simulink model "modello_simulink"  (R2019b)
settings: Solver=VariableStepAuto  StartTime=0.0  StopTime=300.0  RelTol=1e-3
values from neighbouring files (symbols this model uses):
  a1 = rho * D^4 * alpha1    (= 0.000388302366464)    [data.m]    (also in simout.mat)
  a2 = -rho * D^3 * alpha2 * (1 - omega)    (= 0.0037030698432)    [data.m]    (also in simout.mat)
  alpha1 = 0.0113    [data.m]    (also in simout.mat)
  alpha2 = -0.0091    [data.m]    (also in simout.mat)
  current = [seaCurrent; 0; 0; 0]    [data.m]    (also in simout.mat = [0 0 0 0 0 0])
  D = diag([])    [D.m]    (also in data.m = 0.076; simout.mat = 0.076)
  dead_zone_limit = 31.5    [data.m]    (also in simout.mat)
  initial = [0 0 0 0 0 0]'    [Plot_verifica_modello.m]    (also in data.m = [0;0;0;0;0;0]; simout.mat = [0 0 0 0 0 0])
  M = [67.0334425707 0 0 0 0 0 0 67.0334425707 0 0 0 0 ... (36 elements, 6x6)]    [M.mat]    (also in Masse.m = M_rb + M_a; simout.mat)
  M_inv = inv(M)    [Masse.m]    (also in simout.mat = [0.0149179269578 0 0 0 0 0 0 0.0149179269578 0 0 0 0 ... (36)
  n_max = 340    [data.m]    (also in simout.mat)
  omega = 0.1    [data.m]    (also in simout.mat)
  pylonCenter = [ 43.723046 ... (first row only)    [missionB.m]    (also in simout.mat = [43.723046 10.396635 0])
  rho = 1030    [data.m]    (also in simout.mat)
  TAM = [B1 B2 B3 B4 B5 B6 B7]    [TAM_matrice.m]    (also in simout.mat = [1 0 0 0 0 0.25 1 0 0 0 0 -0.25 ... (42 elements, 6x7)])
settings Model: Creator=andrea  LastModifiedBy=Fabio
settings DebuggingCC: ArithmeticOperatorsInVariantConditions=warning
settings SFSimCC: CustomCodeUndefinedFunction=UseInterfaceOnly

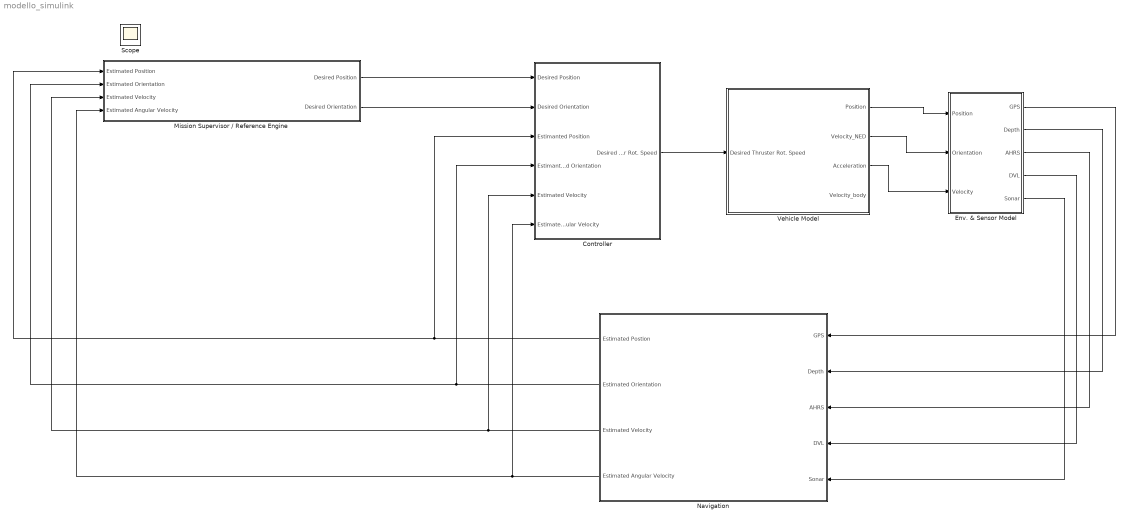
== system modello_simulink ==
  Controller : Subsystem
  Env. & Sensor Model : Subsystem
  Mission Supervisor / Reference Engine : Subsystem
  Navigation : Subsystem
  Vehicle Model : Subsystem
      mask Display: image('maronn.jpg'); % Use "Edit Image" on toolstrip to change.
  Scope : Scope
  wires:
  Mission Supervisor / Reference Engine/1(Desired Position) -> Controller/1(Desired Position)
  Mission Supervisor / Reference Engine/2(Desired Orientation) -> Controller/2(Desired Orientation)
  Controller/1(Desired Thruster Rot. Speed) -> Vehicle Model/1(Desired Thruster Rot. Speed)
  Vehicle Model/1(Position) -> Env. & Sensor Model/1(Position)
  Vehicle Model/2(Velocity_NED) -> Env. & Sensor Model/2(Orientation)
  Vehicle Model/3(Acceleration) -> Env. & Sensor Model/3(Velocity)
  Env. & Sensor Model/1(GPS) -> Navigation/1(GPS)
  Env. & Sensor Model/2(Depth) -> Navigation/2(Depth)
  Env. & Sensor Model/3(AHRS) -> Navigation/3(AHRS)
  Env. & Sensor Model/4(DVL) -> Navigation/4(DVL)
  Env. & Sensor Model/5(Sonar) -> Navigation/5(Sonar)
  Navigation/1(Estimated Postion) -> Controller/3(Estimanted Position), Mission Supervisor / Reference Engine/1(Estimated Position)
  Navigation/2(Estimated Orientation) -> Mission Supervisor / Reference Engine/2(Estimated Orientation), Controller/4(Estimanted Orientation)
  Navigation/3(Estimated Velocity) -> Mission Supervisor / Reference Engine/3(Estimated Velocity), Controller/5(Estimated Velocity)
  Navigation/4(Estimated Angular Velocity) -> Mission Supervisor / Reference Engine/4(Estimated Angular Velocity), Controller/6(Estimated Angular Velocity)

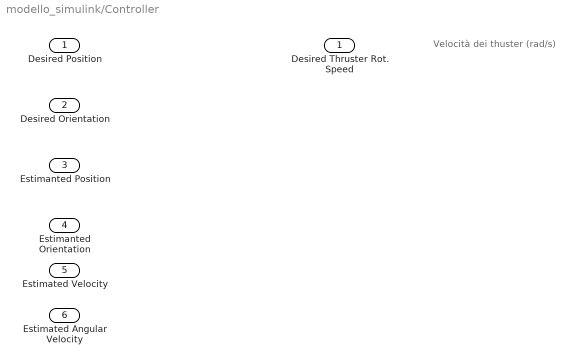
== system modello_simulink/Controller ==
  note: Velocità dei thuster (rad/s)
  Desired Position : Inport
  Desired Orientation : Inport  Port=2
  Estimanted Position : Inport  Port=3
  Estimanted Orientation : Inport  Port=4
  Estimated Velocity : Inport  Port=5
  Estimated Angular Velocity : Inport  Port=6
  Desired Thruster Rot. Speed : Outport

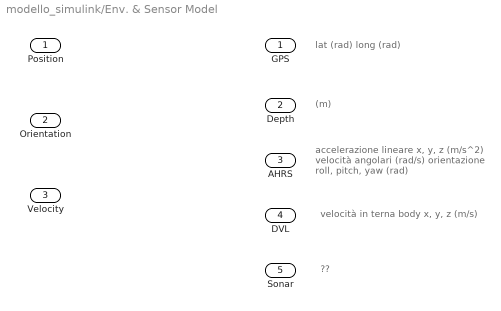
== system modello_simulink/Env. & Sensor Model ==
  note: ??
  note: velocità in terna body x, y, z (m/s)
  note: accelerazione lineare x, y, z (m/s^2)
      | velocità angolari (rad/s)
      | orientazione roll, pitch, yaw (rad)
  note: (m)
  note: lat (rad)
      | long (rad)
  Position : Inport
  Orientation : Inport  Port=2
  Velocity : Inport  Port=3
  GPS : Outport
  Depth : Outport  Port=2
  AHRS : Outport  Port=3
  DVL : Outport  Port=4
  Sonar : Outport  Port=5

== system modello_simulink/Mission Supervisor // Reference Engine ==
  note: Roll (rad): 0 == aligned with water surface
      | Pitch (rad): 0 == aligned with water surface
      | Yaw (rad): 0 == north
  note: Latitude (rad)
      | Longitude (rad)
      | Depth (m): 0 == water surface
  note: Latitude (rad)
      | Longitude (rad)
      | Depth (m): 0 == water surface
  note: Roll (rad): 0 == aligned with water surface
      | Pitch (rad): 0 == aligned with water surface
      | Yaw (rad): 0 == north
  note: Velocity body frame - x, y, z (m/s)
  note: Inertial Frame
      | Roll Rate (rad/s)
      | Pitch Rate (rad/s)
      | Yaw Rate (rad/s)
  Estimated Position : Inport
  Estimated Orientation : Inport  Port=2
  Estimated Velocity : Inport  Port=3
  Estimated Angular Velocity : Inport  Port=4
  Desired Position : Outport
  Desired Orientation : Outport  Port=2

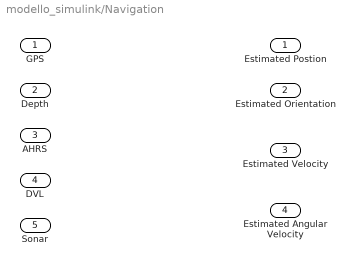
== system modello_simulink/Navigation ==
  GPS : Inport
  Depth : Inport  Port=2
  AHRS : Inport  Port=3
  DVL : Inport  Port=4
  Sonar : Inport  Port=5
  Estimated Postion : Outport
  Estimated Orientation : Outport  Port=2
  Estimated Velocity : Outport  Port=3
  Estimated Angular Velocity : Outport  Port=4

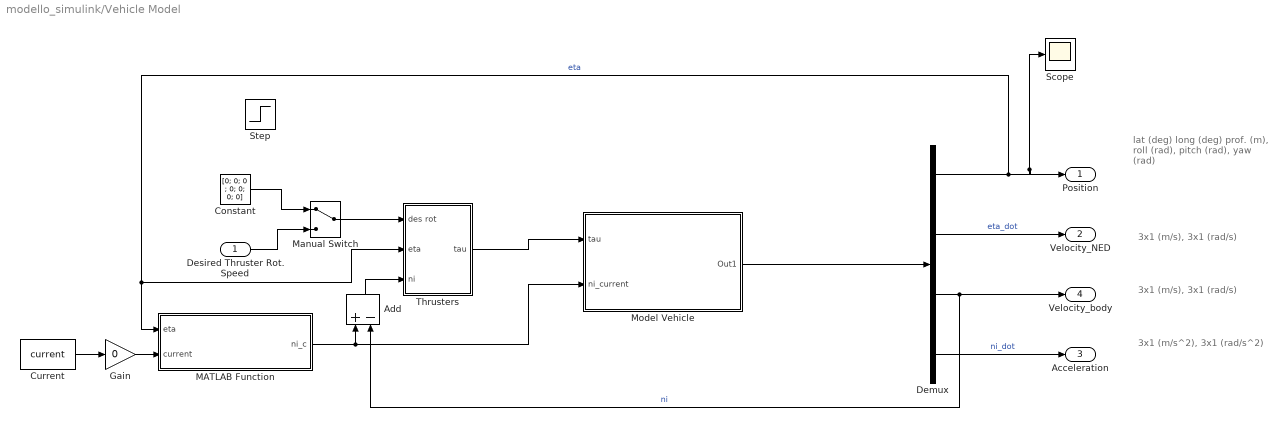
== system modello_simulink/Vehicle Model ==
  note: 3x1 (m/s^2),
      | 3x1 (rad/s^2)
  note: 3x1 (m/s),
      | 3x1 (rad/s)
  note: lat (deg)
      | long (deg)
      | prof. (m),
      | roll (rad),
      | pitch (rad),
      | yaw (rad)
  note: 3x1 (m/s),
      | 3x1 (rad/s)
  Desired Thruster Rot. Speed : Inport
  Add : Sum  Inputs=+-
  Constant : Constant  Value=[0; 0; 0 ; 0; 0; 0; 0]
  Current : Constant  Value=current
  Demux : Demux
  Gain : Gain  Gain=0
  MATLAB Function : MATLAB Function  TreatAsAtomicUnit=on
  Manual Switch : ManualSwitch
  Model Vehicle : Subsystem
      mask Display: image('anna.jpg'); % Use "Edit Image" on toolstrip to change.
  Scope : Scope
  Step : Step  Time=100  Before=[0;0;0;0;-100;-100;-200]  After=[0;0;0;0;0;0;0]  SampleTime=0
  Thrusters : Subsystem
  Position : Outport
  Velocity_NED : Outport  Port=2
  Acceleration : Outport  Port=3
  Velocity_body : Outport  Port=4
  wires:
  Demux/3 -> Velocity_body/1, Add/2  "ni"
  Model Vehicle/1(Out1) -> Demux/1
  Demux/1 -> Thrusters/2(eta), MATLAB Function/1(eta), Position/1, Scope/1  "eta"
  Desired Thruster Rot. Speed/1 -> Manual Switch/2
  Manual Switch/1 -> Thrusters/1(des rot)
  Current/1 -> Gain/1
  Gain/1 -> MATLAB Function/2(current)
  Demux/2 -> Velocity_NED/1  "eta_dot"
  Demux/4 -> Acceleration/1  "ni_dot"
  Thrusters/1(tau) -> Model Vehicle/1(tau)
  Constant/1 -> Manual Switch/1
  MATLAB Function/1(ni_c) -> Model Vehicle/2(ni_current), Add/1
  Add/1 -> Thrusters/3(ni)

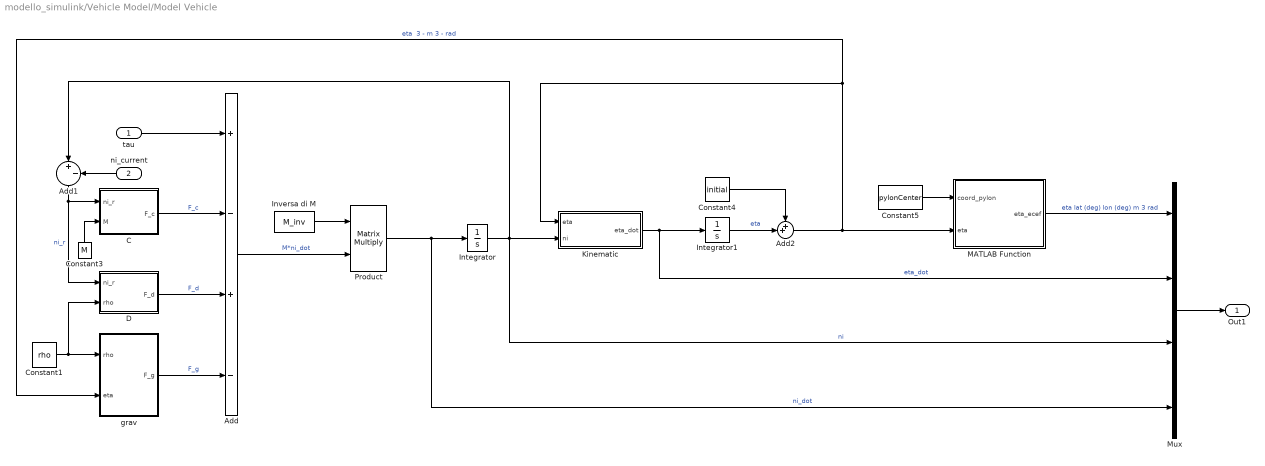
== system modello_simulink/Vehicle Model/Model Vehicle ==
  tau : Inport
  ni_current : Inport  Port=2
  Add : Sum  Inputs=+-+-
  Add1 : Sum  Inputs=|+-
  Add2 : Sum  Inputs=++|
  C : MATLAB Function  TreatAsAtomicUnit=on
  Constant1 : Constant  Value=rho
  Constant3 : Constant  Value=M
  Constant4 : Constant  Value=initial
  Constant5 : Constant  Value=pylonCenter
  D : MATLAB Function  TreatAsAtomicUnit=on
  Integrator : Integrator
  Integrator1 : Integrator
  Inversa di M : Constant  Value=M_inv
  Kinematic : Subsystem
  MATLAB Function : MATLAB Function  TreatAsAtomicUnit=on
  Mux : Mux
  Product : Product  Multiplication=Matrix(*)
  grav : MATLAB Function  TreatAsAtomicUnit=on
  Out1 : Outport  VectorParamsAs1DForOutWhenUnconnected=off
  wires:
  tau/1 -> Add/1
  Product/1 -> Mux/4, Integrator/1  "ni_dot"
  Integrator/1 -> Mux/3, Kinematic/2(ni), Add1/1  "ni"
  ni_current/1 -> Add1/2
  Add1/1 -> D/1(ni_r), C/1(ni_r)  "ni_r"
  Mux/1 -> Out1/1
  C/1(F_c) -> Add/2  "F_c"
  grav/1(F_g) -> Add/4  "F_g"
  Kinematic/1(eta_dot) -> Mux/2, Integrator1/1  "eta_dot"
  Inversa di M/1 -> Product/1
  Add/1 -> Product/2  "M*ni_dot"
  Constant1/1 -> grav/1(rho), D/2(rho)
  Constant3/1 -> C/2(M)
  D/1(F_d) -> Add/3  "F_d"
  Add2/1 -> MATLAB Function/2(eta), grav/2(eta), Kinematic/1(eta)  "eta  3 - m 3 - rad"
  MATLAB Function/1(eta_ecef) -> Mux/1  "eta lat (deg) lon (deg) m 3 rad"
  Constant5/1 -> MATLAB Function/1(coord_pylon)
  Constant4/1 -> Add2/1
  Integrator1/1 -> Add2/2  "eta"

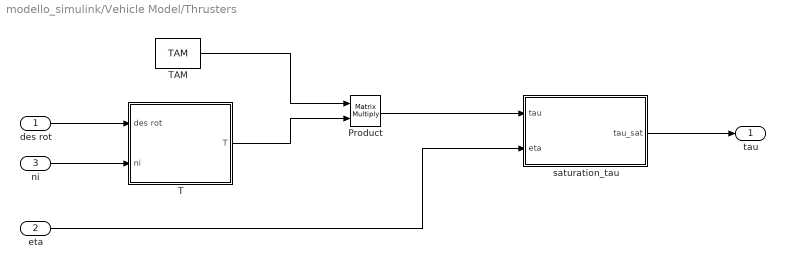
== system modello_simulink/Vehicle Model/Thrusters ==
  des rot : Inport
  eta : Inport  Port=2
  ni : Inport  Port=3
  Product : Product  Multiplication=Matrix(*)
  T : Subsystem
  TAM : Constant  Value=TAM
  saturation_tau : MATLAB Function  TreatAsAtomicUnit=on
  tau : Outport  VectorParamsAs1DForOutWhenUnconnected=off
  wires:
  Product/1 -> saturation_tau/1(tau)
  des rot/1 -> T/1(des rot)
  TAM/1 -> Product/1
  T/1(T) -> Product/2
  saturation_tau/1(tau_sat) -> tau/1
  ni/1 -> T/2(ni)
  eta/1 -> saturation_tau/2(eta)

== system modello_simulink/Vehicle Model/Model Vehicle/Kinematic ==
  eta : Inport
  ni : Inport  Port=2
  Jac : MATLAB Function  TreatAsAtomicUnit=on
  Product : Product  Multiplication=Matrix(*)
  eta_dot : Outport  VectorParamsAs1DForOutWhenUnconnected=off
  wires:
  ni/1 -> Product/2
  Jac/1(J) -> Product/1
  eta/1 -> Jac/1(eta)
  Product/1 -> eta_dot/1

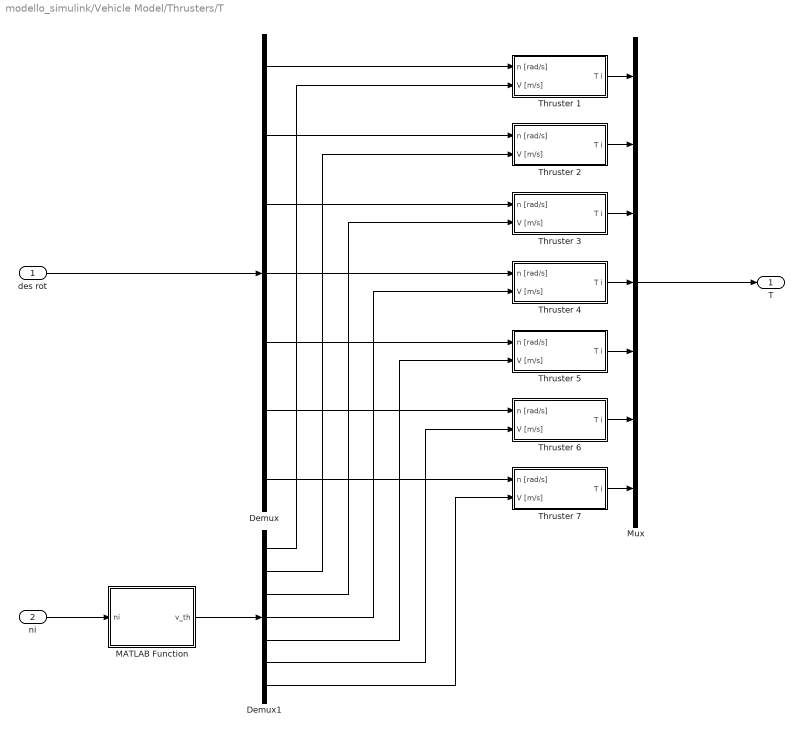
== system modello_simulink/Vehicle Model/Thrusters/T ==
  des rot : Inport
  ni : Inport  Port=2
  Demux : Demux  Outputs=7
  Demux1 : Demux  Outputs=7
  MATLAB Function : MATLAB Function  TreatAsAtomicUnit=on
  Mux : Mux  Inputs=7
  Thruster 1 : Subsystem
  Thruster 2 : Subsystem
  Thruster 3 : Subsystem
  Thruster 4 : Subsystem
  Thruster 5 : Subsystem
  Thruster 6 : Subsystem
  Thruster 7 : Subsystem
  T : Outport  VectorParamsAs1DForOutWhenUnconnected=off
  wires:
  Demux/1 -> Thruster 1/1(n [rad/s])
  Demux/2 -> Thruster 2/1(n [rad/s])
  Demux/3 -> Thruster 3/1(n [rad/s])
  Demux/4 -> Thruster 4/1(n [rad/s])
  Demux/5 -> Thruster 5/1(n [rad/s])
  Demux/6 -> Thruster 6/1(n [rad/s])
  Demux/7 -> Thruster 7/1(n [rad/s])
  des rot/1 -> Demux/1
  Thruster 7/1(T i) -> Mux/7
  Thruster 6/1(T i) -> Mux/6
  Thruster 5/1(T i) -> Mux/5
  Thruster 4/1(T i) -> Mux/4
  Thruster 3/1(T i) -> Mux/3
  Thruster 2/1(T i) -> Mux/2
  Thruster 1/1(T i) -> Mux/1
  Mux/1 -> T/1
  MATLAB Function/1(v_th) -> Demux1/1
  Demux1/1 -> Thruster 1/2(V [m/s])
  Demux1/2 -> Thruster 2/2(V [m/s])
  Demux1/3 -> Thruster 3/2(V [m/s])
  Demux1/4 -> Thruster 4/2(V [m/s])
  Demux1/5 -> Thruster 5/2(V [m/s])
  Demux1/6 -> Thruster 6/2(V [m/s])
  Demux1/7 -> Thruster 7/2(V [m/s])
  ni/1 -> MATLAB Function/1(ni)

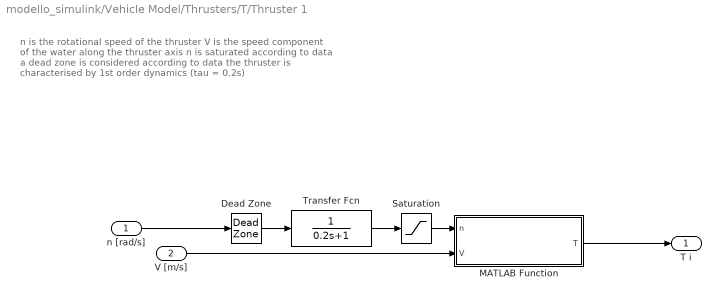
== system modello_simulink/Vehicle Model/Thrusters/T/Thruster 1 ==
  note: n is the rotational speed of the thruster
      | V is the speed component of the water along the thruster axis
      |
      | n is saturated according to data
      | a dead zone is considered according to data
      | the thruster is characterised by 1st order dynamics (tau = 0.2s)
  n [rad/s] : Inport
  V [m/s] : Inport  Port=2
  Dead Zone : DeadZone  LowerValue=-dead_zone_limit  UpperValue=dead_zone_limit  SaturateOnIntegerOverflow=on
  MATLAB Function : MATLAB Function  TreatAsAtomicUnit=on
  Saturation : Saturate  UpperLimit=n_max  LowerLimit=-n_max
  Transfer Fcn : TransferFcn  Denominator=[0.2 1]
  T i : Outport
  wires:
  V [m/s]/1 -> MATLAB Function/2(V)
  Saturation/1 -> MATLAB Function/1(n)
  Transfer Fcn/1 -> Saturation/1
  Dead Zone/1 -> Transfer Fcn/1
  n [rad/s]/1 -> Dead Zone/1
  MATLAB Function/1(T) -> T i/1

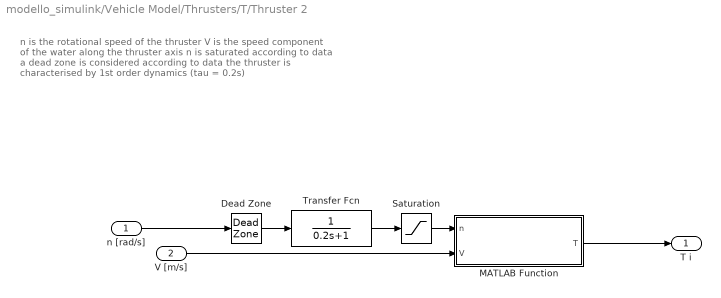
== system modello_simulink/Vehicle Model/Thrusters/T/Thruster 2 ==
  note: n is the rotational speed of the thruster
      | V is the speed component of the water along the thruster axis
      |
      | n is saturated according to data
      | a dead zone is considered according to data
      | the thruster is characterised by 1st order dynamics (tau = 0.2s)
  n [rad/s] : Inport
  V [m/s] : Inport  Port=2
  Dead Zone : DeadZone  LowerValue=-dead_zone_limit  UpperValue=dead_zone_limit  SaturateOnIntegerOverflow=on
  MATLAB Function : MATLAB Function  TreatAsAtomicUnit=on
  Saturation : Saturate  UpperLimit=n_max  LowerLimit=-n_max
  Transfer Fcn : TransferFcn  Denominator=[0.2 1]
  T i : Outport
  wires:
  V [m/s]/1 -> MATLAB Function/2(V)
  Saturation/1 -> MATLAB Function/1(n)
  Transfer Fcn/1 -> Saturation/1
  Dead Zone/1 -> Transfer Fcn/1
  n [rad/s]/1 -> Dead Zone/1
  MATLAB Function/1(T) -> T i/1

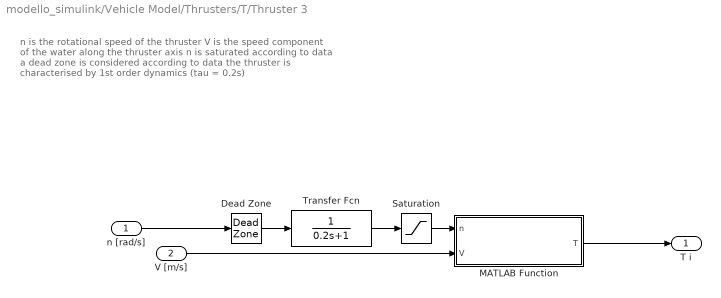
== system modello_simulink/Vehicle Model/Thrusters/T/Thruster 3 ==
  note: n is the rotational speed of the thruster
      | V is the speed component of the water along the thruster axis
      |
      | n is saturated according to data
      | a dead zone is considered according to data
      | the thruster is characterised by 1st order dynamics (tau = 0.2s)
  n [rad/s] : Inport
  V [m/s] : Inport  Port=2
  Dead Zone : DeadZone  LowerValue=-dead_zone_limit  UpperValue=dead_zone_limit  SaturateOnIntegerOverflow=on
  MATLAB Function : MATLAB Function  TreatAsAtomicUnit=on
  Saturation : Saturate  UpperLimit=n_max  LowerLimit=-n_max
  Transfer Fcn : TransferFcn  Denominator=[0.2 1]
  T i : Outport
  wires:
  V [m/s]/1 -> MATLAB Function/2(V)
  Saturation/1 -> MATLAB Function/1(n)
  Transfer Fcn/1 -> Saturation/1
  Dead Zone/1 -> Transfer Fcn/1
  n [rad/s]/1 -> Dead Zone/1
  MATLAB Function/1(T) -> T i/1

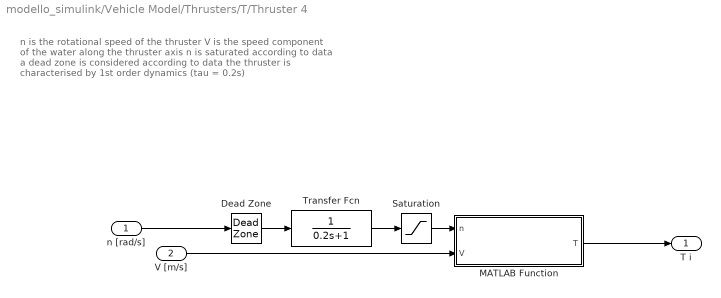
== system modello_simulink/Vehicle Model/Thrusters/T/Thruster 4 ==
  note: n is the rotational speed of the thruster
      | V is the speed component of the water along the thruster axis
      |
      | n is saturated according to data
      | a dead zone is considered according to data
      | the thruster is characterised by 1st order dynamics (tau = 0.2s)
  n [rad/s] : Inport
  V [m/s] : Inport  Port=2
  Dead Zone : DeadZone  LowerValue=-dead_zone_limit  UpperValue=dead_zone_limit  SaturateOnIntegerOverflow=on
  MATLAB Function : MATLAB Function  TreatAsAtomicUnit=on
  Saturation : Saturate  UpperLimit=n_max  LowerLimit=-n_max
  Transfer Fcn : TransferFcn  Denominator=[0.2 1]
  T i : Outport
  wires:
  V [m/s]/1 -> MATLAB Function/2(V)
  Saturation/1 -> MATLAB Function/1(n)
  Transfer Fcn/1 -> Saturation/1
  Dead Zone/1 -> Transfer Fcn/1
  n [rad/s]/1 -> Dead Zone/1
  MATLAB Function/1(T) -> T i/1

== system modello_simulink/Vehicle Model/Thrusters/T/Thruster 5 ==
  note: n is the rotational speed of the thruster
      | V is the speed component of the water along the thruster axis
      |
      | n is saturated according to data
      | a dead zone is considered according to data
      | the thruster is characterised by 1st order dynamics (tau = 0.2s)
  n [rad/s] : Inport
  V [m/s] : Inport  Port=2
  Dead Zone : DeadZone  LowerValue=-dead_zone_limit  UpperValue=dead_zone_limit  SaturateOnIntegerOverflow=on
  MATLAB Function : MATLAB Function  TreatAsAtomicUnit=on
  Saturation : Saturate  UpperLimit=n_max  LowerLimit=-n_max
  Transfer Fcn : TransferFcn  Denominator=[0.2 1]
  T i : Outport
  wires:
  V [m/s]/1 -> MATLAB Function/2(V)
  Saturation/1 -> MATLAB Function/1(n)
  Transfer Fcn/1 -> Saturation/1
  Dead Zone/1 -> Transfer Fcn/1
  n [rad/s]/1 -> Dead Zone/1
  MATLAB Function/1(T) -> T i/1

== system modello_simulink/Vehicle Model/Thrusters/T/Thruster 6 ==
  note: n is the rotational speed of the thruster
      | V is the speed component of the water along the thruster axis
      |
      | n is saturated according to data
      | a dead zone is considered according to data
      | the thruster is characterised by 1st order dynamics (tau = 0.2s)
  n [rad/s] : Inport
  V [m/s] : Inport  Port=2
  Dead Zone : DeadZone  LowerValue=-dead_zone_limit  UpperValue=dead_zone_limit  SaturateOnIntegerOverflow=on
  MATLAB Function : MATLAB Function  TreatAsAtomicUnit=on
  Saturation : Saturate  UpperLimit=n_max  LowerLimit=-n_max
  Transfer Fcn : TransferFcn  Denominator=[0.2 1]
  T i : Outport
  wires:
  V [m/s]/1 -> MATLAB Function/2(V)
  Saturation/1 -> MATLAB Function/1(n)
  Transfer Fcn/1 -> Saturation/1
  Dead Zone/1 -> Transfer Fcn/1
  n [rad/s]/1 -> Dead Zone/1
  MATLAB Function/1(T) -> T i/1

== system modello_simulink/Vehicle Model/Thrusters/T/Thruster 7 ==
  note: n is the rotational speed of the thruster
      | V is the speed component of the water along the thruster axis
      |
      | n is saturated according to data
      | a dead zone is considered according to data
      | the thruster is characterised by 1st order dynamics (tau = 0.2s)
  n [rad/s] : Inport
  V [m/s] : Inport  Port=2
  Dead Zone : DeadZone  LowerValue=-dead_zone_limit  UpperValue=dead_zone_limit  SaturateOnIntegerOverflow=on
  MATLAB Function : MATLAB Function  TreatAsAtomicUnit=on
  Saturation : Saturate  UpperLimit=n_max  LowerLimit=-n_max
  Transfer Fcn : TransferFcn  Denominator=[0.2 1]
  T i : Outport
  wires:
  V [m/s]/1 -> MATLAB Function/2(V)
  Saturation/1 -> MATLAB Function/1(n)
  Transfer Fcn/1 -> Saturation/1
  Dead Zone/1 -> Transfer Fcn/1
  n [rad/s]/1 -> Dead Zone/1
  MATLAB Function/1(T) -> T i/1

== matlab function modello_simulink/Vehicle Model/Model Vehicle/D ==
  data: ni_r input; F_d output; rho input
function F_d = D_forces(ni_r, rho)
    ni_lin = ni_r(1:3);
    ni_ang = ni_r(4:6);
    a = 0.35;
    b = a;
    c = 0.19;
    A_ab = pi*a*b;      % moto lin lungo z; rotatorio intorno a x e y
    A_bc = pi*b*c;      % moto lin lungo x; rotatorio intorno a z
    A_ac = pi*a*c;      % moto lin lungo y
%     C_d  =  0.0489;
%     D_coeff = -1/2*rho*C_d*diag([A_bc, A_ac, A_ab, A_bc, A_ac, A_ab]);
%     F_d = D_coeff*(abs(ni_r).*ni_r);
    visc = 0.001;       % Pa*s (per una temperatura di 20° e rho = 1030)
    vmax = 0.3;
    Di = 0.7;
    Re = Di/(visc/rho)*vmax; % Re = 2*1e5
    Cd = 0.49;
    rm_z = 4*c/(3*pi);
    rm_xy = 4*a/(3*pi);
    D_lin = -1/2*rho*Cd*diag([A_bc, A_ac, A_ab])*(abs(ni_lin).*ni_lin);
    D_ang = -1/2*rho*Cd*diag([rm_xy^3*A_ab, rm_xy^3*A_ab, rm_z^3*A_bc])*(abs(ni_ang).*ni_ang);
    F_d = [D_lin; D_ang];
end

== matlab function modello_simulink/Vehicle Model/Model Vehicle/C ==
  data: ni_r input; F_c output; M input
function F_c = C(ni_r, M)
    ni = ni_r;
    M11 = M(1:3,1:3);
    M22 = M(4:6,4:6);
    ni1 = ni(1:3);
    ni2 = ni(4:6);
    C11 = zeros(3,3);
    s1 = M11*ni1;
    C12 = - [0 -s1(3) s1(2); s1(3) 0 -s1(1); -s1(2) s1(1) 0];
    C21 = C12;
    s2 = M22*ni2;
    C22 = - [0 -s2(3) s2(2); s2(3) 0 -s2(1); -s2(2) s2(1) 0];
    F_c = [C11 C12; C21 C22]*ni_r;
end

== matlab function modello_simulink/Vehicle Model/Model Vehicle/grav ==
  data: rho input; eta input; F_g output
function F_g = grav(rho, eta)
    eta2 = eta(4:6);
    g = 9.81;   
    a = 0.35;
    b = a;
    c = 0.19;
    massa = 100;
    if eta(3) >= c
       V = 4/3*pi*a*b*c;
    else
       V = 4/3*pi*a*b*c - (pi*a*b/(3*c^2))*((eta(3)-c)^2)*(3*c - abs(eta(3) - c)); 
    end
    W = massa*g;
    B = rho*V*g;
    J = Jac(eta2);
    J1 = J(1:3,1:3);
    J2 = J(4:6,4:6);
    f_g = inv(J1)*[0; 0; W];
    f_b = inv(J1)*[0; 0; -B];
    r_g = [0; 0; 0];
    r_b = [0; 0; -c/2];
    %TODO: inserire un contributo nullo di forza quando siamo a galla (?)
%     if eta(3) < 0
%        F_g = [0; 0; 0; 0; 0; 0];
%     else
    F_g = -[f_g + f_b; cross(r_g,f_g) + cross(r_b,f_b)];
%     end
end

== matlab function modello_simulink/Vehicle Model/Model Vehicle/Kinematic/Jac ==
  data: eta input; J output
function J = Jac(eta)
    eta2 = eta(4:6);
    phi = eta2(1);
    theta = eta2(2);
    psi = eta2(3);
    Rx = [1 0 0; 0 cos(phi) sin(phi); 0 -sin(phi) cos(phi)];
    Ry = [cos(theta) 0 -sin(theta); 0 1 0; sin(theta) 0 cos(theta)];
    Rz = [cos(psi) sin(psi) 0; -sin(psi) cos(psi) 0; 0 0 1];
    J1 = Rz'*Ry'*Rx';
    J2 = [1 sin(phi)*tan(theta) cos(phi)*tan(theta); ...
        0 cos(phi) -sin(phi); ...
        0 sin(phi)/cos(theta) cos(phi)/cos(theta)];
    J = blkdiag(J1, J2);
end

== matlab function modello_simulink/Vehicle Model/Thrusters/T/Thruster 1/MATLAB Function ==
  data: n input; T output; V input; D parameter; omega parameter; a1 parameter; a2 parameter; alpha1 parameter; alpha2 parameter
function T = thrusterModel(n, V, D, omega, a1, a2, alpha1, alpha2)

Va = (1-omega) * V;     % Advancement velocity at the propeller
J0 = Va/(n*D);          % Advancement Coefficient

if J0 > -alpha1/alpha2  % Out of linearity domain (right side)
    T = 0;              % A null generated thrust is assumed
    
elseif J0 < 0           % Out of linearity domain (left side)
    T = a1*abs(n)*n;    % Bollard thrust is assumed

else                    % Within the linearity domain
    T = a1*abs(n)*n - a2*abs(n)*V;
end

== matlab function modello_simulink/Vehicle Model/Thrusters/T/Thruster 2/MATLAB Function ==
  data: n input; T output; V input; D parameter; omega parameter; a1 parameter; a2 parameter; alpha1 parameter; alpha2 parameter
function T = thrusterModel(n, V, D, omega, a1, a2, alpha1, alpha2)

Va = (1-omega) * V;     % Advancement velocity at the propeller
J0 = Va/(n*D);          % Advancement Coefficient

if J0 > -alpha1/alpha2  % Out of linearity domain (right side)
    T = 0;              % A null generated thrust is assumed
    
elseif J0 < 0           % Out of linearity domain (left side)
    T = a1*abs(n)*n;    % Bollard thrust is assumed

else                    % Within the linearity domain
    T = a1*abs(n)*n - a2*abs(n)*V;
end

== matlab function modello_simulink/Vehicle Model/Thrusters/T/Thruster 3/MATLAB Function ==
  data: n input; T output; V input; D parameter; omega parameter; a1 parameter; a2 parameter; alpha1 parameter; alpha2 parameter
function T = thrusterModel(n, V, D, omega, a1, a2, alpha1, alpha2)

Va = (1-omega) * V;     % Advancement velocity at the propeller
J0 = Va/(n*D);          % Advancement Coefficient

if J0 > -alpha1/alpha2  % Out of linearity domain (right side)
    T = 0;              % A null generated thrust is assumed
    
elseif J0 < 0           % Out of linearity domain (left side)
    T = a1*abs(n)*n;    % Bollard thrust is assumed

else                    % Within the linearity domain
    T = a1*abs(n)*n - a2*abs(n)*V;
end

== matlab function modello_simulink/Vehicle Model/Thrusters/T/Thruster 4/MATLAB Function ==
  data: n input; T output; V input; D parameter; omega parameter; a1 parameter; a2 parameter; alpha1 parameter; alpha2 parameter
function T = thrusterModel(n, V, D, omega, a1, a2, alpha1, alpha2)

Va = (1-omega) * V;     % Advancement velocity at the propeller
J0 = Va/(n*D);          % Advancement Coefficient

if J0 > -alpha1/alpha2  % Out of linearity domain (right side)
    T = 0;              % A null generated thrust is assumed
    
elseif J0 < 0           % Out of linearity domain (left side)
    T = a1*abs(n)*n;    % Bollard thrust is assumed

else                    % Within the linearity domain
    T = a1*abs(n)*n - a2*abs(n)*V;
end

== matlab function modello_simulink/Vehicle Model/Thrusters/T/Thruster 5/MATLAB Function ==
  data: n input; T output; V input; D parameter; omega parameter; a1 parameter; a2 parameter; alpha1 parameter; alpha2 parameter
function T = thrusterModel(n, V, D, omega, a1, a2, alpha1, alpha2)

Va = (1-omega) * V;     % Advancement velocity at the propeller
J0 = Va/(n*D);          % Advancement Coefficient

if J0 > -alpha1/alpha2  % Out of linearity domain (right side)
    T = 0;              % A null generated thrust is assumed
    
elseif J0 < 0           % Out of linearity domain (left side)
    T = a1*abs(n)*n;    % Bollard thrust is assumed

else                    % Within the linearity domain
    T = a1*abs(n)*n - a2*abs(n)*V;
end

== matlab function modello_simulink/Vehicle Model/Thrusters/T/Thruster 6/MATLAB Function ==
  data: n input; T output; V input; D parameter; omega parameter; a1 parameter; a2 parameter; alpha1 parameter; alpha2 parameter
function T = thrusterModel(n, V, D, omega, a1, a2, alpha1, alpha2)

Va = (1-omega) * V;     % Advancement velocity at the propeller
J0 = Va/(n*D);          % Advancement Coefficient

if J0 > -alpha1/alpha2  % Out of linearity domain (right side)
    T = 0;              % A null generated thrust is assumed
    
elseif J0 < 0           % Out of linearity domain (left side)
    T = a1*abs(n)*n;    % Bollard thrust is assumed

else                    % Within the linearity domain
    T = a1*abs(n)*n - a2*abs(n)*V;
end

== matlab function modello_simulink/Vehicle Model/Thrusters/T/Thruster 7/MATLAB Function ==
  data: n input; T output; V input; D parameter; omega parameter; a1 parameter; a2 parameter; alpha1 parameter; alpha2 parameter
function T = thrusterModel(n, V, D, omega, a1, a2, alpha1, alpha2)

Va = (1-omega) * V;     % Advancement velocity at the propeller
J0 = Va/(n*D);          % Advancement Coefficient

if J0 > -alpha1/alpha2  % Out of linearity domain (right side)
    T = 0;              % A null generated thrust is assumed
    
elseif J0 < 0           % Out of linearity domain (left side)
    T = a1*abs(n)*n;    % Bollard thrust is assumed

else                    % Within the linearity domain
    T = a1*abs(n)*n - a2*abs(n)*V;
end

== matlab function modello_simulink/Vehicle Model/Model Vehicle/MATLAB Function ==
  data: coord_pylon input; eta input; eta_ecef output
function eta_ecef = nedToEcef(coord_pylon, eta)

    coder.extrinsic('wgs84Ellipsoid');

    coder.extrinsic('ned2geodetic');
    
    eta_pos = eta(1:6);
    wgs84 = wgs84Ellipsoid('meter'); %TODO verificare che esprima le coordinate nello stesso modo dell'ECEF dato in missionB.m
    [eta_pos(1), eta_pos(2)] = ned2geodetic(eta(1), eta(2), eta(3), coord_pylon(1), coord_pylon(2), coord_pylon(3), wgs84,'degrees');
    
    eta_pos(3) = eta(3);
    eta_pos(4:6) = eta_pos(4:6);
    
    eta_ecef = eta_pos;
    
end

== matlab function modello_simulink/Vehicle Model/MATLAB Function ==
  data: eta input; ni_c output; current input
function ni_c = current_ned2body(eta, current)
    eta2 = eta(4:6)*pi/180;     % eta2 espresso in radianti
    ni_c = Jac(eta2)'*current;
end

== matlab function modello_simulink/Vehicle Model/Thrusters/T/MATLAB Function ==
  data: ni input; v_th output
function v_th = thrusters(ni)
p1 = [-0.35 -0.25 0]';
p2 = [-0.35 0.25 0]';
p3 = [-0.25 -0.35 0]';
p4 = [0.25 0.35 0]';
p5 = [-0.25 -0.25 -0.19]';
p6 = [-0.25 0.25 -0.19]';
p7 = [0.25 0 -0.19]';

t1 = [1 0 0]';
t2 = t1;
t3 = [0 1 0]';
t4 = -t3;
t5 = [0 0 1]';
t6 = t5;
t7 = t5;

v_lin = ni(1:3);
v_ang = ni(4:6);

vp1 = v_lin + cross(v_ang, p1);
vp2 = v_lin + cross(v_ang, p2);
vp3 = v_lin + cross(v_ang, p3);
vp4 = v_lin + cross(v_ang, p4);
vp5 = v_lin + cross(v_ang, p5);
vp6 = v_lin + cross(v_ang, p6);
vp7 = v_lin + cross(v_ang, p7);

v1 = vp1'*t1;
v2 = vp2'*t2;
v3 = vp3'*t3;
v4 = vp4'*t4;
v5 = vp5'*t5;
v6 = vp6'*t6;
v7 = vp7'*t7;

v_th = [ v1 v2 v3 v4 v5 v6 v7]';
end

== matlab function modello_simulink/Vehicle Model/Thrusters/saturation_tau ==
  data: tau input; tau_sat output; eta input
function tau_sat = sat_tau(tau, eta)
    tau_sat = [0;0;0;0;0;0];
    tau_sat = tau;

    if eta(3) < 0.19 %semiasse c
        tau_sat(3) = 0;
    end
    
end
